simulink model "lss"  (R2022b)
settings: Solver=FixedStepAuto  StartTime=0.0  StopTime=Inf  FixedStep=0.001  RelTol=1e-3  EnableMultiTasking=on
InitFcn:
  | clear mex
model workspace (MAT data in the model file):
  worldsim_instance : object (value not decoded)
values from neighbouring files (symbols this model uses):
  ADAS_Control_Mode = 1    [LSS_parameters.m]    (also in lss_ini_param.sldd = 1.0)
  butter_a = 1.0 -1.9911142922016536 0.99115359586893548    [lss_ini_param.sldd]
  butter_a_lka_out = 1.0 -1.5610180758007179 0.641351538057563    [lss_ini_param.sldd]
  butter_b = 9.825916820482009E-6 1.9651833640964018E-5 9.825916820482009E-6    [lss_ini_param.sldd]
  butter_b_lka_out = 0.020083365564211246 0.040166731128422492 0.020083365564211246    [lss_ini_param.sldd]
  index_variant_approaching_speed = 3.0    [lss_ini_param.sldd]
  initCond = vi_worldsim_load_scenario(worldsim_process,scenario_path,'lss_online')    [launcher.m]
  LDW_Activity_Flag = 1    [LSS_parameters.m]    (also in lss_ini_param.sldd = 1.0)
  LDW_Freq_Hz = Sensor_Freq_worldsim    [LSS_parameters.m]    (also in lss_ini_param.sldd = 50.0)
  LDW_LaneGap_dydt_Warning = 50    [LSS_parameters.m]    (also in lss_ini_param.sldd = 50.0)
  LDW_LaneGap_Warning = [0.5 0.25]    [LSS_parameters.m]    (also in lss_ini_param.sldd = 0.5 0.25)
  LDW_Min_Speed = 60    [LSS_parameters.m]    (also in lss_ini_param.sldd = 60.0)
  LDW_Steer_Vibration_Amplitude = 5    [LSS_parameters.m]    (also in lss_ini_param.sldd = 5.0)
  LDW_Steer_Vibration_Freq = 25    [LSS_parameters.m]    (also in lss_ini_param.sldd = 25.0)
  LKA_Activity_Flag = 1    [LSS_parameters.m]    (also in lss_ini_param.sldd = 1.0)
  LKA_D = [0.2 0.3]    [LSS_parameters.m]    (also in lss_ini_param.sldd = 0.2 0.3)
  LKA_Dyn_Rate_Limiter_Gain = 0.1    [LSS_parameters.m]    (also in lss_ini_param.sldd)
  LKA_Dyn_Rate_Limiter_Power = 10    [LSS_parameters.m]    (also in lss_ini_param.sldd = 10.0)
  LKA_Error_dydt_Off = 1    [LSS_parameters.m]    (also in lss_ini_param.sldd = 1.0)
  LKA_Error_Max = 3    [LSS_parameters.m]    (also in lss_ini_param.sldd = 3.0)
  LKA_Error_Off = 0.5    [LSS_parameters.m]    (also in lss_ini_param.sldd)
  LKA_Freq_Hz = Sensor_Freq_worldsim    [LSS_parameters.m]    (also in lss_ini_param.sldd = 50.0)
  LKA_I = [0.025 0.05]    [LSS_parameters.m]    (also in lss_ini_param.sldd = 0.025 0.05)
  LKA_Lane_Gap_Activate = [0.25 0.125]    [LSS_parameters.m]    (also in lss_ini_param.sldd = -0.05 0.125)
  LKA_Lane_Gap_dydt_Activate = 50    [LSS_parameters.m]    (also in lss_ini_param.sldd = 50.0)
  LKA_Min_Speed = 60    [LSS_parameters.m]    (also in lss_ini_param.mat = 50; lss_ini_param.sldd = 50.0)
  LKA_On_Display_Freq = 5    [LSS_parameters.m]    (also in lss_ini_param.sldd = 5.0)
  LKA_P = [0.1 0.2]    [LSS_parameters.m]    (also in lss_ini_param.sldd = 0.1 0.2)
  LKA_Steer_Rate_Max_radps = 1    [LSS_parameters.m]    (also in lss_ini_param.sldd = 1.0)
  radar_source = 2    [LSS_parameters.m]    (also in lss_ini_param.sldd = 2.0)
  Sensor_Freq_worldsim = 50    [launcher.m]    (also in lss_ini_param.sldd = 50.0)
  simulation_crt = '../VI-CarRealTime_model/SedanCar_WorldSim_Offline_send_svm.xml'    [launcher.m]
  stop_number_collisions = 5    [launcher.m]
  stop_speed = 0.001    [launcher.m]
  stop_time = 20    [launcher.m]
  target_speed = 72    [LSS_parameters.m]    (also in launcher.m = initCond.initialVelocity * 3.6)
  variant_approaching_speed = v_lat    [launcher.m]    (also in lss_ini_param.sldd = 0.2 0.3 0.4 0.5 0.6)
  vehicle_width = 1.86    [LSS_parameters.m]    (also in lss_ini_param.sldd = 2.05)
undefined symbols (not defined in the file or in its folder): Driver_Demands, light_brake_center, light_brake_left, light_brake_right, steer_assist, vicrt_initcallback, vicrt_initmexcallback, vicrt_simulationmanager
libraries: simulink x39, simwbSfunlib x15, viworldsim_lib x5
(part 2 of 6)

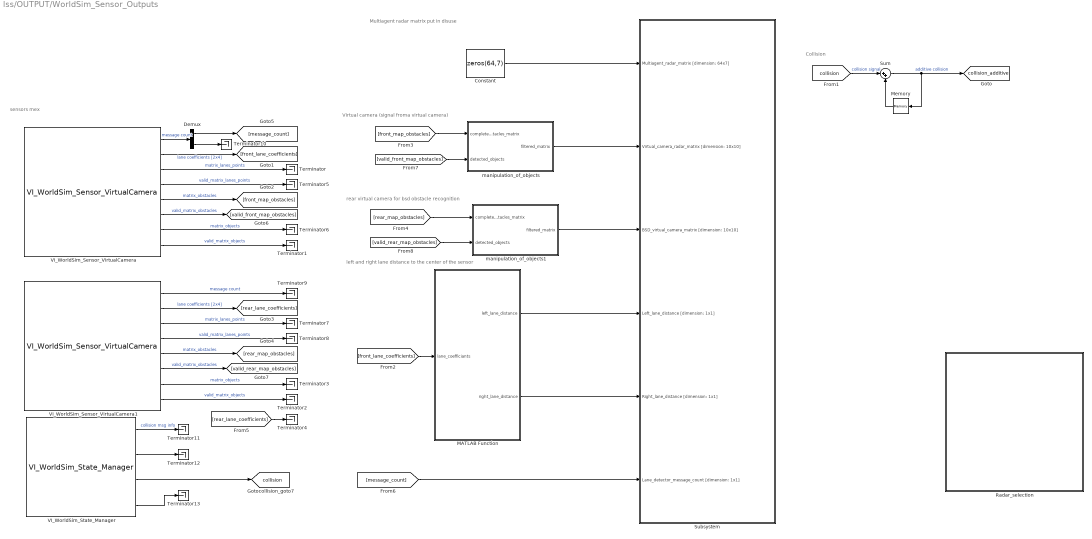
== system lss/OUTPUT/WorldSim_Sensor_Outputs ==
  note: Collision
  note: left and right lane distance to the center of the sensor
  note: Virtual camera (signal froma virtual camera)
  note: Multiagent radar matrix
      | put in disuse
  note: rear virtual camera for bsd obstacle recognition
  note: sensors mex
  Constant : Constant  Value=zeros(64,7)
  Demux : Demux  Outputs=2
  MATLAB Function : MATLAB Function  TreatAsAtomicUnit=on
  Memory : Memory  InheritSampleTime=on
  Radar_selection : Subsystem
  Subsystem : Subsystem
  Sum : Sum  Inputs=|++
  Terminator{,1..13} (14 alike) : Terminator
  VI_WorldSim_Sensor_VirtualCamera : viworldsim_lib/VI-WorldSim Sensors/VI_WorldSim_Sensor_VirtualCamera  worldsim_endpoint_ip=worldsim_instance.endpoint_ip  worldsim_endpoint_port=worldsim_instance.endpoint_port  worldsim_car_name='ego'  worldsim_sensor_name='Front_VirtualCam'  max_lanes=10  max_obstacles=10  worldsim_verbose=off
  VI_WorldSim_Sensor_VirtualCamera1 : viworldsim_lib/VI-WorldSim Sensors/VI_WorldSim_Sensor_VirtualCamera  worldsim_endpoint_ip=worldsim_instance.endpoint_ip  worldsim_endpoint_port=worldsim_instance.endpoint_port  worldsim_car_name='ego'  worldsim_sensor_name='Rear_VirtualCam'  max_lanes=10  max_obstacles=10  worldsim_verbose=off
  VI_WorldSim_State_Manager : viworldsim_lib/VI-WorldSim Sensors/VI_WorldSim_State_Manager  worldsim_endpoint_ip=worldsim_instance.endpoint_ip  worldsim_endpoint_port=worldsim_instance.endpoint_port  worldsim_car_name='ego'  worldsim_verbose=off
  manipulation_of_objects : MATLAB Function  TreatAsAtomicUnit=on
  manipulation_of_objects1 : MATLAB Function  TreatAsAtomicUnit=on
  tag scope: collision=global, collision_additive=global
  wires:
  Sum/1 -> Memory/1, [collision_additive]  "additive collision"
  [collision] -> Sum/1  "collision signal"
  Memory/1 -> Sum/2
  MATLAB Function/1(left_lane_distance) -> Subsystem/4(Left_lane_distance [dimension: 1x1])
  [message_count] -> Subsystem/6(Lane_detector_message_count [dimension: 1x1])
  manipulation_of_objects1/1(filtered_matrix) -> Subsystem/3(BSD_virtual_camera_matrix [dimension: 10x10])
  manipulation_of_objects/1(filtered_matrix) -> Subsystem/2(Virtual_camera_radar_matrix [dimension: 10x10])
  Constant/1 -> Subsystem/1(Multiagent_radar_matrix [dimension: 64x7])
  [valid_rear_map_obstacles] -> manipulation_of_objects1/2(detected_objects)
  MATLAB Function/2(right_lane_distance) -> Subsystem/5(Right_lane_distance [dimension: 1x1])
  [front_lane_coefficients] -> MATLAB Function/1(lane_coefficiants)
  [rear_map_obstacles] -> manipulation_of_objects1/1(complete_obstacles_matrix)
  [valid_front_map_obstacles] -> manipulation_of_objects/2(detected_objects)
  [front_map_obstacles] -> manipulation_of_objects/1(complete_obstacles_matrix)
  VI_WorldSim_Sensor_VirtualCamera/1 -> Demux/1  "message count"
  VI_WorldSim_State_Manager/1 -> Terminator11/1  "collision msg info"
  VI_WorldSim_Sensor_VirtualCamera/8 -> Terminator1/1  "valid_matrix_objects"
  VI_WorldSim_Sensor_VirtualCamera/5 -> [front_map_obstacles]  "matrix_obstacles"
  VI_WorldSim_Sensor_VirtualCamera/4 -> Terminator5/1  "valid_matrix_lanes_points"
  VI_WorldSim_Sensor_VirtualCamera/6 -> [valid_front_map_obstacles]  "valid_matrix_obstacles"
  VI_WorldSim_Sensor_VirtualCamera1/2 -> [rear_lane_coefficients]  "lane coefficients [2x4]"
  VI_WorldSim_Sensor_VirtualCamera/3 -> Terminator/1  "matrix_lanes_points"
  VI_WorldSim_Sensor_VirtualCamera1/1 -> Terminator9/1  "message count"
  VI_WorldSim_Sensor_VirtualCamera1/7 -> Terminator3/1  "matrix_objects"
  VI_WorldSim_Sensor_VirtualCamera1/8 -> Terminator2/1  "valid_matrix_objects"
  VI_WorldSim_Sensor_VirtualCamera/7 -> Terminator6/1  "matrix_objects"
  VI_WorldSim_Sensor_VirtualCamera/2 -> [front_lane_coefficients]  "lane coefficients [2x4]"
  VI_WorldSim_Sensor_VirtualCamera1/4 -> Terminator8/1  "valid_matrix_lanes_points"
  VI_WorldSim_State_Manager/3 -> [collision]
  VI_WorldSim_Sensor_VirtualCamera1/3 -> Terminator7/1  "matrix_lanes_points"
  [rear_lane_coefficients] -> Terminator4/1
  Demux/2 -> Terminator10/1
  VI_WorldSim_Sensor_VirtualCamera1/5 -> [rear_map_obstacles]  "matrix_obstacles"
  VI_WorldSim_Sensor_VirtualCamera1/6 -> [valid_rear_map_obstacles]  "valid_matrix_obstacles"
  Demux/1 -> [message_count]
  VI_WorldSim_State_Manager/2 -> Terminator12/1
  VI_WorldSim_State_Manager/4 -> Terminator13/1

== system lss/OUTPUT/rough data reporting ==
  Cast To Double : DataTypeConversion  OutDataTypeStr=double  SaturateOnIntegerOverflow=off  RndMeth=Floor
  Cast To Double1 : DataTypeConversion  OutDataTypeStr=double  SaturateOnIntegerOverflow=off  RndMeth=Floor
  Clock : Clock
  Compare To Constant : simulink/Logic and Bit Operations/Compare To Constant  relop=<=  const=0.0  OutDataTypeStr=boolean
  Compare To Constant1 : simulink/Logic and Bit Operations/Compare To Constant  relop=<=  const=0.0  OutDataTypeStr=boolean
  Compare To Constant2 : simulink/Logic and Bit Operations/Compare To Constant  relop=>  const=0.1  OutDataTypeStr=boolean
  Product : Product
  Scope LDW_Steering_Torque_in_out : Scope  NumInputPorts=2
  Sum1 : Sum
  To Workspace : ToWorkspace  VariableName=number_collision  SampleTime=-1
      settings: Save2DSignal=2-D array (concatenate along first dimension)
  To Workspace1 : ToWorkspace  VariableName=longitudinal_accelerations  SampleTime=-1
      settings: Save2DSignal=2-D array (concatenate along first dimension)
  To Workspace2 : ToWorkspace  VariableName=lateral_accelerations  SampleTime=-1
      settings: Save2DSignal=2-D array (concatenate along first dimension)
  To Workspace3 : ToWorkspace  VariableName=crossed_lanes  SampleTime=-1
      settings: Save2DSignal=2-D array (concatenate along first dimension)
  wires:
  Clock/1 -> Compare To Constant2/1
  Compare To Constant1/1 -> Cast To Double1/1
  [Lateral_Accelerations] -> To Workspace2/1
  [LaneGap_right_ws] -> Compare To Constant1/1
  Cast To Double/1 -> Sum1/1
  Compare To Constant2/1 -> Product/2
  [collision_additive] -> To Workspace/1
  Compare To Constant/1 -> Cast To Double/1
  [Longitudinal_Accelerations] -> To Workspace1/1
  [LaneGap_left_ws] -> Compare To Constant/1
  Product/1 -> To Workspace3/1
  Cast To Double1/1 -> Sum1/2
  Sum1/1 -> Product/1
  [Steering_feedback_torque] -> Scope LDW_Steering_Torque_in_out/2  "Output Steering Wheel Torque"
  [LDW_Steering_Torque] -> Scope LDW_Steering_Torque_in_out/1  "LDW Additional Steering Assist torque"

== system lss/VI-CarRealTime/Input_Bus ==
  Driver_Demands.str_swa : Inport
  steer_assist.torque : Inport  Port=2
  Driver_Demands.throttle : Inport  Port=3
  Driver_Demands.clutch : Inport  Port=4
  Driver_Demands.brake : Inport  Port=5
  Driver_Demands.gear : Inport  Port=6
  Bus2Map : Subsystem
  Inputs : Subsystem
  VicrtBusAssignment : BusAssignment  AssignedSignals=Driver_Demands.str_swa,steer_assist.torque,Driver_Demands.throttle,Driver_Demands.clutch,Driver_Demands.brake,Driver_Demands.gear
  vicrt input : Outport
  wires:
  Bus2Map/1(Map Out) -> vicrt input/1
  VicrtBusAssignment/1 -> Bus2Map/1(Bus In)
  Inputs/1(Inputs) -> VicrtBusAssignment/1  "Inputs"
  Driver_Demands.str_swa/1 -> VicrtBusAssignment/2
  steer_assist.torque/1 -> VicrtBusAssignment/3
  Driver_Demands.throttle/1 -> VicrtBusAssignment/4
  Driver_Demands.clutch/1 -> VicrtBusAssignment/5
  Driver_Demands.brake/1 -> VicrtBusAssignment/6
  Driver_Demands.gear/1 -> VicrtBusAssignment/7

== system lss/VI-CarRealTime/Output_Bus ==
  Outputs : Inport
  IOmap2bus : Subsystem
  VicrtBusSelector : BusSelector  OutputSignals=aero_forces,Brake,bul_jounce_stop_data,bul_rebound_stop_data,bur_jounce_stop_data,bur_rebound_stop_data,bus_dmp_jounce_stop_data,bus_ins_jounce_stop_data,bus_roll_dmp_jounce_stop_data,bus_spr_jounce_stop_data,chassis_accelerations,chassis_displacements,chassis_velocities,clutch,condition_sensors,cross_weight,dal_ride_damper_data,Damper,dar_ride_damper_data,das_ride_damper_data,das_roll_damper_data,das_third_damper_data,differential_central,differential_front,differential_rear,differential_speeds,differential_torques,driver_demands,driving_machine_monitor,engine,fuel_consumption,ges_chassis_XFORM,Gyro,Hook_rear,Inerter,inl_ride_inerter_data,inr_ride_inerter_data,ins_inerter_data,jfs_torsional_stiffness_data,Jounce_Bumper,nsl_ride_spring_data,nsr_ride_spring_data,nss_ride_spring_data,Rebound_Bumper,res_dmp_rebound_stop_data,res_ins_rebound_stop_data,res_roll_dmp_rebound_stop_data,res_spr_rebound_stop_data,rhl_front_setup_sensor_data,rhl_rear_setup_sensor_data,rhr_front_setup_sensor_data,rhr_rear_setup_sensor_data,rhs_front_setup_sensor_data,rhs_rear_setup_sensor_data,Road,Sensor,Spring,Steering_System,Suspension,System,System_Mass_Center,til_wheel_tire_forces,til_wheel_tire_kinematics,til_wheel_tire_rolling_states,Tire,tir_wheel_tire_forces,tir_wheel_tire_kinematics,tir_wheel_tire_rolling_states,torque_converter,transmission,ues_third_spring_data,upright_accelerometer,Vehicle,Vehicle_States,Wheel,wheel_angles,whl_front_wheel_XFORM,whl_rear_wheel_XFORM,whl_twin_rear_wheel_XFORM,whr_front_wheel_XFORM,whr_rear_wheel_XFORM,whr_twin_rear_wheel_XFORM,Steering_Column,Steering_Torsion_Bar,Steering_Rack_Pinion,Motor,path_sensor,Animator_Widget,ges_hub_XFORMFL,hub2cp_XFORMFL,cp_force_longitudinalFL,cp_force_lateralFL,cp_force_normalFL,ges_hub_XFORMFR,hub2cp_XFORMFR,cp_force_longitudinalFR,cp_force_lateralFR,cp_force_normalFR,ges_hub_XFORMRL,hub2cp_XFORMRL,cp_force_longitudinalRL,cp_force_lateralRL,cp_force_normalRL,ges_hub_XFORMRR,hub2cp_XFORMRR,cp_force_longitudinalRR,cp_force_lateralRR,cp_force_normalRR,Road_Material  OutputAsBus=on
  adapter : Subsystem
  OutputBus : Outport  VectorParamsAs1DForOutWhenUnconnected=off
  wires:
  IOmap2bus/1(Out) -> VicrtBusSelector/1
  Outputs/1 -> IOmap2bus/1(In)
  VicrtBusSelector/1 -> adapter/1(inputBus)
  adapter/1(outputBus) -> OutputBus/1

== system lss/VI-CarRealTime/vicrt_mex Standard ==
  In1 : Inport
  vicrt_mex : S-Function  InitFcn=vicrt_initmexcallback(gcb);  FunctionName=vicrt_mex  Parameters=vicrt_inputfile,vicrt_outprefix,AniFlag,intStep,inpPortDim,outPortDim,NoDirectFeedthrough,AuxDataStruct,inpPortVecSize,outPortVecSize  SFunctionDeploymentMode=off  EnableBusSupport=off
  Out1 : Outport
  wires:
  In1/1 -> vicrt_mex/1
  vicrt_mex/1 -> Out1/1

== system lss/VI-WorldSim Lights Manager/Lights ==
  light_brake_left : Inport
  light_brake_right : Inport  Port=2
  light_brake_center : Inport  Port=3
  Bus Selector : BusSelector  OutputSignals=light_low_beam_left,light_low_beam_right,light_high_beam_left,light_high_beam_right,light_indicator_left,light_indicator_right,light_fog_left,light_fog_right,light_tail_left,light_tail_right,light_brake_left,light_brake_right,light_brake_center,light_reverse,light_daytime
  Default Lights Bus : Subsystem
  LightsBusAssignment : BusAssignment  AssignedSignals=light_brake_left,light_brake_right,light_brake_center
  Mux : Mux  Inputs=15
  Out1 : Outport  VectorParamsAs1DForOutWhenUnconnected=off
  wires:
  LightsBusAssignment/1 -> Bus Selector/1
  Bus Selector/5 -> Mux/5  "<light_indicator_left>"
  Default Lights Bus/1(Out1) -> LightsBusAssignment/1
  Bus Selector/11 -> Mux/11  "<light_brake_left>"
  Bus Selector/10 -> Mux/10  "<light_tail_right>"
  Bus Selector/2 -> Mux/2  "<light_low_beam_right>"
  Bus Selector/9 -> Mux/9  "<light_tail_left>"
  Bus Selector/12 -> Mux/12  "<light_brake_right>"
  Mux/1 -> Out1/1
  Bus Selector/8 -> Mux/8  "<light_fog_right>"
  Bus Selector/14 -> Mux/14  "<light_reverse>"
  Bus Selector/4 -> Mux/4  "<light_high_beam_right>"
  Bus Selector/3 -> Mux/3  "<light_high_beam_left>"
  Bus Selector/15 -> Mux/15  "<light_daytime>"
  Bus Selector/13 -> Mux/13  "<light_brake_center>"
  Bus Selector/6 -> Mux/6  "<light_indicator_right>"
  Bus Selector/1 -> Mux/1  "<light_low_beam_left>"
  Bus Selector/7 -> Mux/7  "<light_fog_left>"
  light_brake_left/1 -> LightsBusAssignment/2
  light_brake_right/1 -> LightsBusAssignment/3
  light_brake_center/1 -> LightsBusAssignment/4

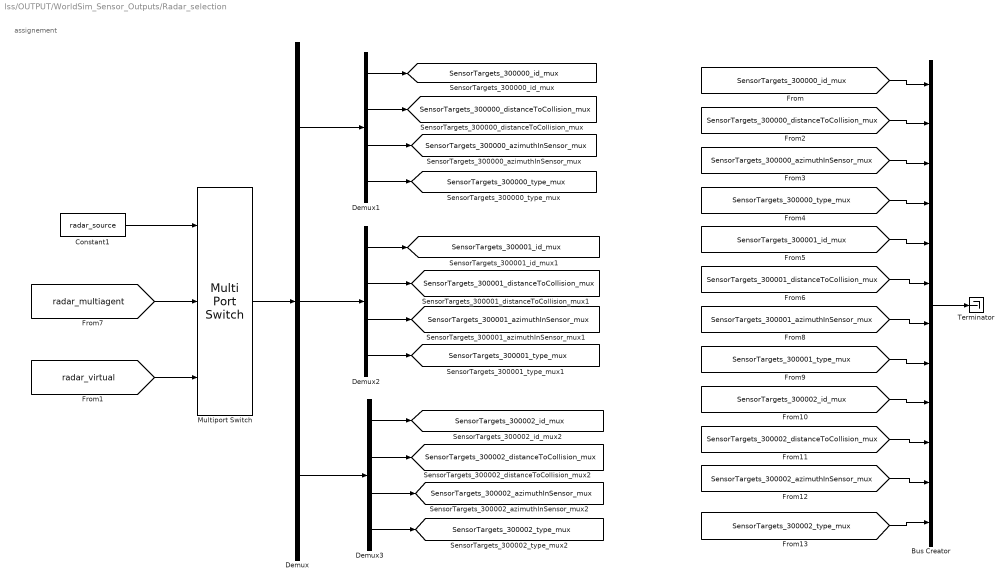
== system lss/OUTPUT/WorldSim_Sensor_Outputs/Radar_selection ==
  note: assignement
  Bus Creator : BusCreator  Inputs=12
  Constant1 : Constant  Value=radar_source
  Demux : Demux  Outputs=3
  Demux1 : Demux
  Demux2 : Demux
  Demux3 : Demux
  Multiport Switch : MultiPortSwitch  Inputs=2  SaturateOnIntegerOverflow=off  InputSameDT=off
  Terminator : Terminator
  tag scope: SensorTargets_300000_azimuthInSensor_mux=global, SensorTargets_300000_distanceToCollision_mux=global, SensorTargets_300000_id_mux=global, SensorTargets_300000_type_mux=global, SensorTargets_300001_azimuthInSensor_mux=global, SensorTargets_300001_distanceToCollision_mux=global, SensorTargets_300001_id_mux=global, SensorTargets_300001_type_mux=global, SensorTargets_300002_azimuthInSensor_mux=global, SensorTargets_300002_distanceToCollision_mux=global, SensorTargets_300002_id_mux=global, SensorTargets_300002_type_mux=global
  wires:
  [radar_virtual] -> Multiport Switch/3
  [radar_multiagent] -> Multiport Switch/2
  Constant1/1 -> Multiport Switch/1
  Multiport Switch/1 -> Demux/1
  Demux1/1 -> [SensorTargets_300000_id_mux]
  Demux3/4 -> [SensorTargets_300002_type_mux]
  Demux3/1 -> [SensorTargets_300002_id_mux]
  Demux1/4 -> [SensorTargets_300000_type_mux]
  Demux3/2 -> [SensorTargets_300002_distanceToCollision_mux]
  Demux2/3 -> [SensorTargets_300001_azimuthInSensor_mux]
  Demux1/2 -> [SensorTargets_300000_distanceToCollision_mux]
  Demux/1 -> Demux1/1
  Demux1/3 -> [SensorTargets_300000_azimuthInSensor_mux]
  Demux2/2 -> [SensorTargets_300001_distanceToCollision_mux]
  Demux3/3 -> [SensorTargets_300002_azimuthInSensor_mux]
  Demux2/4 -> [SensorTargets_300001_type_mux]
  Demux/3 -> Demux3/1
  Demux/2 -> Demux2/1
  Demux2/1 -> [SensorTargets_300001_id_mux]
  [SensorTargets_300000_id_mux] -> Bus Creator/1
  [SensorTargets_300000_distanceToCollision_mux] -> Bus Creator/2
  [SensorTargets_300000_azimuthInSensor_mux] -> Bus Creator/3
  [SensorTargets_300000_type_mux] -> Bus Creator/4
  [SensorTargets_300001_id_mux] -> Bus Creator/5
  [SensorTargets_300001_distanceToCollision_mux] -> Bus Creator/6
  [SensorTargets_300001_azimuthInSensor_mux] -> Bus Creator/7
  [SensorTargets_300001_type_mux] -> Bus Creator/8
  [SensorTargets_300002_id_mux] -> Bus Creator/9
  [SensorTargets_300002_distanceToCollision_mux] -> Bus Creator/10
  [SensorTargets_300002_azimuthInSensor_mux] -> Bus Creator/11
  [SensorTargets_300002_type_mux] -> Bus Creator/12
  Bus Creator/1 -> Terminator/1

== system lss/OUTPUT/WorldSim_Sensor_Outputs/Subsystem ==
  Multiagent_radar_matrix [dimension: 64x7] : Inport
  Virtual_camera_radar_matrix [dimension: 10x10] : Inport  Port=2
  BSD_virtual_camera_matrix [dimension: 10x10] : Inport  Port=3
  Left_lane_distance [dimension: 1x1] : Inport  Port=4
  Right_lane_distance [dimension: 1x1] : Inport  Port=5
  Lane_detector_message_count [dimension: 1x1] : Inport  Port=6
  Semitrack : Constant  Value=vehicle_width/2
  Terminator : Terminator
  Terminator1 : Terminator
  bsd setection from ostacle recognition : Subsystem
  lane marking acquisition : Subsystem
  "multiagent radar SimpleRadar_... are single double representing id, yaw, range, power_db, range_rate, yaw_rate, status" : Subsystem
  "obstacle detection " : Subsystem
  tag scope: frame_worldsim_left=global, frame_worldsim_right=global
  wires:
  Semitrack/1 -> lane marking acquisition/1(Semitrack), bsd setection from ostacle recognition/1(semitrack)
  Virtual_camera_radar_matrix [dimension: 10x10]/1 -> "obstacle detection "/1(Virtual_camera_obstacle_matrix)
  BSD_virtual_camera_matrix [dimension: 10x10]/1 -> bsd setection from ostacle recognition/2(BSD_matrix_obstalces)
  Left_lane_distance [dimension: 1x1]/1 -> lane marking acquisition/2(Left_lane_marking)
  Right_lane_distance [dimension: 1x1]/1 -> lane marking acquisition/3(Right_lane_marking)
  Multiagent_radar_matrix [dimension: 64x7]/1 -> "multiagent radar SimpleRadar_... are single double representing id, yaw, range, power_db, range_rate, yaw_rate, status"/1(Virtual_radar_obstacle_matrix)
  Lane_detector_message_count [dimension: 1x1]/1 -> [frame_worldsim_right], [frame_worldsim_left]
  [frame_worldsim_left] -> Terminator/1
  [frame_worldsim_right] -> Terminator1/1

== system lss/VI-CarRealTime/Input_Bus/Bus2Map ==
  Bus In : Inport
  Bus Selector : BusSelector  OutputSignals=Driver_Demands.str_swa,Subsystem_Activation.Internal_Steering_Column_Activity,Driver_Demands.rack_displacement,Driver_Demands.throttle,Driver_Demands.gear,Driver_Demands.clutch,Driver_Demands.brake,Driver_Demands.target_speed,Driver_Demands.target_acc,Brake_System_General.brk_mast_cyl_pres,Brake_System_General.brk_bias_front,ABS.Internal_ABS_Activity,ABS.ABS_threshold,Driver_Demands.user_maneuver_ID,Driver_Demands.user_input_steering,Driver_Demands.user_input_throttle,Driver_Demands.user_input_braking,Driver_Demands.user_input_gear,Driver_Demands.user_input_clutch,TCS.Internal_TCS_Activity,TCS.TCS_threshold,Friction.tire_mu.L1,Friction.tire_mu.L2,Friction.tire_mu.R1,Friction.tire_mu.R2,Subsystem_Activation.Internal_Brake_System_Activity.L1,Brake_System.brk_mmag_sign.L1,Brake_System.brk_mmag_unsign.L1,Brake_System.brk_pres.L1,Brake_System.brk_pres_gain.L1,Brake_System.brk_mu.L1,Subsystem_Activation.Internal_Brake_System_Activity.L2,Brake_System.brk_mmag_sign.L2,Brake_System.brk_mmag_unsign.L2,Brake_System.brk_pres.L2,Brake_System.brk_pres_gain.L2,Brake_System.brk_mu.L2,Subsystem_Activation.Internal_Brake_System_Activity.R1,Brake_System.brk_mmag_sign.R1,Brake_System.brk_mmag_unsign.R1,Brake_System.brk_pres.R1,Brake_System.brk_pres_gain.R1,Brake_System.brk_mu.R1,Subsystem_Activation.Internal_Brake_System_Activity.R2,Brake_System.brk_mmag_sign.R2,Brake_System.brk_mmag_unsign.R2,Brake_System.brk_pres.R2,Brake_System.brk_pres_gain.R2,Brake_System.brk_mu.R2,Hook.Fx.rear,Hook.Fy.rear,Hook.Fz.rear,Hook.Mx.rear,Hook.My.rear,Hook.Mz.rear,Rear_Steering_Actuator_disp.str_swa.left,Rear_Steering_Actuator_disp.str_swa.right,Steering.steer_at_spindle.L1,Steering.steer_at_spindle.L2,Steering.steer_at_spindle.R1,Steering.steer_at_spindle.R2,Steering.Internal_Hand_Wheel_Torque_Computation,Steering.Hand_Wheel_Torque,Subsystem_Activation.Internal_Clutch_Activity,Subsystem_Activation.Internal_Engine_Activity,Subsystem_Activation.Internal_Engine_Idle_MaxRev_Controls_Activity,Subsystem_Activation.Internal_Gearbox_Activity,Subsystem_Activation.Internal_CentralDifferential_Activity,Subsystem_Activation.Internal_FrontDifferential_Activity,Subsystem_Activation.Internal_RearDifferential_Activity,Engine.engine_omega,Engine.engine_max_trq,Engine.engine_min_trq,Engine.engine_trq,Engine.clutch_inputplate_torque,Engine.non_termic_engine_trq,Engine.efficiency,Engine.throttle_scaling,Engine.control_mode,Engine.throttle_offset,Clutch.clutch_trq,Clutch.gearbox_inputshaft_torque,Clutch.inputplate_angle,Clutch.inputplate_omega,Clutch.inputplate_alpha,Clutch.efficiency,Differential_Central.efficiency,Differential_Central.diff_front_inputshaft_torque,Differential_Central.diff_rear_inputshaft_torque,Differential_Central.gearbox_outputshaft_angle,Differential_Central.gearbox_outputshaft_omega,Differential_Central.gearbox_outputshaft_alpha,Differential_Front.efficiency,Differential_Front.wheel_front_left_torque,Differential_Front.wheel_front_right_torque,Differential_Front.diff_central_front_outputshaft_angle,Differential_Front.diff_central_front_outputshaft_omega,Differential_Front.diff_central_front_outputshaft_alpha,Differential_Rear.efficiency,Differential_Rear.wheel_rear_left_torque,Differential_Rear.wheel_rear_right_torque,Differential_Rear.diff_central_rear_outputshaft_angle,Differential_Rear.diff_central_rear_outputshaft_omega,Differential_Rear.diff_central_rear_outputshaft_alpha,Antiroll_Bar.activity_flag.front,Antiroll_Bar.activity_flag.rear,Antiroll_Bar.force.front,Antiroll_Bar.force.rear,Wheel_driving.moment.L1,Wheel_driving.moment.L2,Wheel_driving.moment.R1,Wheel_driving.moment.R2,Subsystem_Activation.Internal_Aero_Activity,Aerodynamic.my_scaling,Aerodynamic.fx_central_scaling,Aerodynamic.fz_front_scaling,Aerodynamic.fz_rear_scaling,Aerodynamic.fx_front,Aerodynamic.fy_front,Aerodynamic.fz_front,Aerodynamic.fx_rear,Aerodynamic.fy_rear,Aerodynamic.fz_rear,Aerodynamic.fx_center,Aerodynamic.fy_center,Aerodynamic.fz_center,Aerodynamic.mx,Aerodynamic.my,Aerodynamic.mz,Irregularity.road.L1,Irregularity.road.L2,Irregularity.road.R1,Irregularity.road.R2,Main_Damper.force.L1,Main_Damper.activity_flag.L1,Main_Damper.force.L2,Main_Damper.activity_flag.L2,Main_Damper.force.R1,Main_Damper.activity_flag.R1,Main_Damper.force.R2,Main_Damper.activity_flag.R2,Main_Spring.force.L1,Main_Spring.activity_flag.L1,Main_Spring.force.L2,Main_Spring.activity_flag.L2,Main_Spring.force.R1,Main_Spring.activity_flag.R1,Main_Spring.force.R2,Main_Spring.activity_flag.R2,Main_Bumpstop.force.L1,Main_Bumpstop.activity_flag.L1,Main_Bumpstop.force.L2,Main_Bumpstop.activity_flag.L2,Main_Bumpstop.force.R1,Main_Bumpstop.activity_flag.R1,Main_Bumpstop.force.R2,Main_Bumpstop.activity_flag.R2,Main_Reboundstop.force.L1,Main_Reboundstop.activity_flag.L1,Main_Reboundstop.force.L2,Main_Reboundstop.activity_flag.L2,Main_Reboundstop.force.R1,Main_Reboundstop.activity_flag.R1,Main_Reboundstop.force.R2,Main_Reboundstop.activity_flag.R2,Auxiliary_vertical.force.L1,Auxiliary_vertical.activity_flag.L1,Auxiliary_vertical.force.L2,Auxiliary_vertical.activity_flag.L2,Auxiliary_vertical.force.R1,Auxiliary_vertical.activity_flag.R1,Auxiliary_vertical.force.R2,Auxiliary_vertical.activity_flag.R2,Main_Inerter.force.L1,Main_Inerter.activity_flag.L1,Main_Inerter.force.L2,Main_Inerter.activity_flag.L2,Main_Inerter.force.R1,Main_Inerter.activity_flag.R1,Main_Inerter.force.R2,Main_Inerter.activity_flag.R2,Third_Element.Damper_force.front,Third_Element.Damper_activity_flag.front,Third_Element.Damper_force.rear,Third_Element.Damper_activity_flag.rear,Third_Element.Spring.front,Third_Element.Spring_activity_flag.front,Third_Element.Spring.rear,Third_Element.Spring_activity_flag.rear,Mono_Element.Damper.front,Mono_Element.Damper_activity_flag.front,Mono_Element.Damper.rear,Mono_Element.Damper_activity_flag.rear,Mono_Element.Inerter.front,Mono_Element.Inerter_activity_flag.front,Mono_Element.Inerter.rear,Mono_Element.Inerter_activity_flag.rear,Mono_Element.Spring.front,Mono_Element.Spring_activity_flag.front,Mono_Element.Spring.rear,Mono_Element.Spring_activity_flag.rear,Mono_Element.Bumpstop_Spring.front,Mono_Element.Bumpstop_Spring_activity_flag.front,Mono_Element.Bumpstop_Spring.rear,Mono_Element.Bumpstop_Spring_activity_flag.rear,Mono_Element.Reboundstop_Spring.front,Mono_Element.Reboundstop_Spring_activity_flag.front,Mono_Element.Reboundstop_Spring.rear,Mono_Element.Reboundstop_Spring_activity_flag.rear,Mono_Element.Bumpstop_Damper.front,Mono_Element.Bumpstop_Damper_activity_flag.front,Mono_Element.Bumpstop_Damper.rear,Mono_Element.Bumpstop_Damper_activity_flag.rear,Mono_Element.Reboundstop_Damper.front,Mono_Element.Reboundstop_Damper_activity_flag.front,Mono_Element.Reboundstop_Damper.rear,Mono_Element.Reboundstop_Damper_activity_flag.rear,Mono_Element.Roll_Damper.front,Mono_Element.Roll_Damper_activity_flag.front,Mono_Element.Roll_Damper.rear,Mono_Element.Roll_Damper_activity_flag.rear,Subsystem_Activation.Tire_Force_x.L1,Subsystem_Activation.Tire_Force_y.L1,Subsystem_Activation.Tire_Force_z.L1,Subsystem_Activation.Tire_Moment_x.L1,Subsystem_Activation.Tire_Moment_y.L1,Subsystem_Activation.Tire_Moment_z.L1,Tire_Force.Fx.L1,Tire_Force.Fy.L1,Tire_Force.Fz.L1,Tire_Moment.Mx.L1,Tire_Moment.My.L1,Tire_Moment.Mz.L1,Subsystem_Activation.Tire_Force_x.L2,Subsystem_Activation.Tire_Force_y.L2,Subsystem_Activation.Tire_Force_z.L2,Subsystem_Activation.Tire_Moment_x.L2,Subsystem_Activation.Tire_Moment_y.L2,Subsystem_Activation.Tire_Moment_z.L2,Tire_Force.Fx.L2,Tire_Force.Fy.L2,Tire_Force.Fz.L2,Tire_Moment.Mx.L2,Tire_Moment.My.L2,Tire_Moment.Mz.L2,Subsystem_Activation.Tire_Force_x.R1,Subsystem_Activation.Tire_Force_y.R1,Subsystem_Activation.Tire_Force_z.R1,Subsystem_Activation.Tire_Moment_x.R1,Subsystem_Activation.Tire_Moment_y.R1,Subsystem_Activation.Tire_Moment_z.R1,Tire_Force.Fx.R1,Tire_Force.Fy.R1,Tire_Force.Fz.R1,Tire_Moment.Mx.R1,Tire_Moment.My.R1,Tire_Moment.Mz.R1,Subsystem_Activation.Tire_Force_x.R2,Subsystem_Activation.Tire_Force_y.R2,Subsystem_Activation.Tire_Force_z.R2,Subsystem_Activation.Tire_Moment_x.R2,Subsystem_Activation.Tire_Moment_y.R2,Subsystem_Activation.Tire_Moment_z.R2,Tire_Force.Fx.R2,Tire_Force.Fy.R2,Tire_Force.Fz.R2,Tire_Moment.Mx.R2,Tire_Moment.My.R2,Tire_Moment.Mz.R2,Ext_Body.force.X,Ext_Body.force.Y,Ext_Body.force.Z,Ext_Body.moment.X,Ext_Body.moment.Y,Ext_Body.moment.Z,Ext_Ground.force.X,Ext_Ground.force.Y,Ext_Ground.force.Z,Ext_Ground.moment.X,Ext_Ground.moment.Y,Ext_Ground.moment.Z,Ext_Tracking.force.X,Ext_Tracking.force.Y,Ext_Tracking.moment.X,Ext_Tracking.moment.Y,steer_assist.force,steer_assist.torque,steering_torque.torque,steering_assist.motor_torque,Steering_System.auxiliary_steering_torque,Steering_System.eps_map,Fuel_Mass.Internal_mass_activation,Fuel_Mass.External_mass,GearBox.efficiency,GearBox.transmission_ratio,GearBox.diff_central_inputshaft_torque,GearBox.clutch_outputplate_angle,GearBox.clutch_outputplate_omega,GearBox.clutch_outputplate_alpha,GearBox.automatic_gearbox_shifting_mode,GearBox.manual_shifting_activity,GearBox.sequential_shifting_activity,Driver_Demands.gear_upshift,Driver_Demands.gear_downshift
  Mux : Mux  Inputs=304
  Map Out : Outport
  wires:
  Mux/1 -> Map Out/1
  Bus In/1 -> Bus Selector/1
  Bus Selector/1 -> Mux/1  "<str_swa>"
  Bus Selector/2 -> Mux/2  "<Internal_Steering_Column_Activity>"
  Bus Selector/3 -> Mux/3  "<rack_displacement>"
  Bus Selector/4 -> Mux/4  "<throttle>"
  Bus Selector/5 -> Mux/5  "<gear>"
  Bus Selector/6 -> Mux/6  "<clutch>"
  Bus Selector/7 -> Mux/7  "<brake>"
  Bus Selector/8 -> Mux/8  "<target_speed>"
  Bus Selector/9 -> Mux/9  "<target_acc>"
  Bus Selector/10 -> Mux/10  "<brk_mast_cyl_pres>"
  Bus Selector/11 -> Mux/11  "<brk_bias_front>"
  Bus Selector/12 -> Mux/12  "<Internal_ABS_Activity>"
  Bus Selector/13 -> Mux/13  "<ABS_threshold>"
  Bus Selector/14 -> Mux/14  "<user_maneuver_ID>"
  Bus Selector/15 -> Mux/15  "<user_input_steering>"
  Bus Selector/16 -> Mux/16  "<user_input_throttle>"
  Bus Selector/17 -> Mux/17  "<user_input_braking>"
  Bus Selector/18 -> Mux/18  "<user_input_gear>"
  Bus Selector/19 -> Mux/19  "<user_input_clutch>"
  Bus Selector/20 -> Mux/20  "<Internal_TCS_Activity>"
  Bus Selector/21 -> Mux/21  "<TCS_threshold>"
  Bus Selector/22 -> Mux/22  "<L1>"
  Bus Selector/23 -> Mux/23  "<L2>"
  Bus Selector/24 -> Mux/24  "<R1>"
  Bus Selector/25 -> Mux/25  "<R2>"
  Bus Selector/26 -> Mux/26  "<L1>"
  Bus Selector/27 -> Mux/27  "<L1>"
  Bus Selector/28 -> Mux/28  "<L1>"
  Bus Selector/29 -> Mux/29  "<L1>"
  Bus Selector/30 -> Mux/30  "<L1>"
  Bus Selector/31 -> Mux/31  "<L1>"
  Bus Selector/32 -> Mux/32  "<L2>"
  Bus Selector/33 -> Mux/33  "<L2>"
  Bus Selector/34 -> Mux/34  "<L2>"
  Bus Selector/35 -> Mux/35  "<L2>"
  Bus Selector/36 -> Mux/36  "<L2>"
  Bus Selector/37 -> Mux/37  "<L2>"
  Bus Selector/38 -> Mux/38  "<R1>"
  Bus Selector/39 -> Mux/39  "<R1>"
  Bus Selector/40 -> Mux/40  "<R1>"
  Bus Selector/41 -> Mux/41  "<R1>"
  Bus Selector/42 -> Mux/42  "<R1>"
  Bus Selector/43 -> Mux/43  "<R1>"
  Bus Selector/44 -> Mux/44  "<R2>"
  Bus Selector/45 -> Mux/45  "<R2>"
  Bus Selector/46 -> Mux/46  "<R2>"
  Bus Selector/47 -> Mux/47  "<R2>"
  Bus Selector/48 -> Mux/48  "<R2>"
  Bus Selector/49 -> Mux/49  "<R2>"
  Bus Selector/50 -> Mux/50  "<rear>"
  Bus Selector/51 -> Mux/51  "<rear>"
  Bus Selector/52 -> Mux/52  "<rear>"
  Bus Selector/53 -> Mux/53  "<rear>"
  Bus Selector/54 -> Mux/54  "<rear>"
  Bus Selector/55 -> Mux/55  "<rear>"
  Bus Selector/56 -> Mux/56  "<left>"
  Bus Selector/57 -> Mux/57  "<right>"
  Bus Selector/58 -> Mux/58  "<L1>"
  Bus Selector/59 -> Mux/59  "<L2>"
  Bus Selector/60 -> Mux/60  "<R1>"
  Bus Selector/61 -> Mux/61  "<R2>"
  Bus Selector/62 -> Mux/62  "<Internal_Hand_Wheel_Torque_Computation>"
  Bus Selector/63 -> Mux/63  "<Hand_Wheel_Torque>"
  Bus Selector/64 -> Mux/64  "<Internal_Clutch_Activity>"
  Bus Selector/65 -> Mux/65  "<Internal_Engine_Activity>"
  Bus Selector/66 -> Mux/66  "<Internal_Engine_Idle_MaxRev_Controls_Activity>"
  Bus Selector/67 -> Mux/67  "<Internal_Gearbox_Activity>"
  Bus Selector/68 -> Mux/68  "<Internal_CentralDifferential_Activity>"
  Bus Selector/69 -> Mux/69  "<Internal_FrontDifferential_Activity>"
  Bus Selector/70 -> Mux/70  "<Internal_RearDifferential_Activity>"
  Bus Selector/71 -> Mux/71  "<engine_omega>"
  Bus Selector/72 -> Mux/72  "<engine_max_trq>"
  Bus Selector/73 -> Mux/73  "<engine_min_trq>"
  Bus Selector/74 -> Mux/74  "<engine_trq>"
  Bus Selector/75 -> Mux/75  "<clutch_inputplate_torque>"
  Bus Selector/76 -> Mux/76  "<non_termic_engine_trq>"
  Bus Selector/77 -> Mux/77  "<efficiency>"
  Bus Selector/78 -> Mux/78  "<throttle_scaling>"
  Bus Selector/79 -> Mux/79  "<control_mode>"
  Bus Selector/80 -> Mux/80  "<throttle_offset>"
  Bus Selector/81 -> Mux/81  "<clutch_trq>"
  Bus Selector/82 -> Mux/82  "<gearbox_inputshaft_torque>"
  Bus Selector/83 -> Mux/83  "<inputplate_angle>"
  Bus Selector/84 -> Mux/84  "<inputplate_omega>"
  Bus Selector/85 -> Mux/85  "<inputplate_alpha>"
  Bus Selector/86 -> Mux/86  "<efficiency>"
  Bus Selector/87 -> Mux/87  "<efficiency>"
  Bus Selector/88 -> Mux/88  "<diff_front_inputshaft_torque>"
  Bus Selector/89 -> Mux/89  "<diff_rear_inputshaft_torque>"
  Bus Selector/90 -> Mux/90  "<gearbox_outputshaft_angle>"
  Bus Selector/91 -> Mux/91  "<gearbox_outputshaft_omega>"
  Bus Selector/92 -> Mux/92  "<gearbox_outputshaft_alpha>"
  Bus Selector/93 -> Mux/93  "<efficiency>"
  Bus Selector/94 -> Mux/94  "<wheel_front_left_torque>"
  Bus Selector/95 -> Mux/95  "<wheel_front_right_torque>"
  Bus Selector/96 -> Mux/96  "<diff_central_front_outputshaft_angle>"
  Bus Selector/97 -> Mux/97  "<diff_central_front_outputshaft_omega>"
  Bus Selector/98 -> Mux/98  "<diff_central_front_outputshaft_alpha>"
  Bus Selector/99 -> Mux/99  "<efficiency>"
  Bus Selector/100 -> Mux/100  "<wheel_rear_left_torque>"
  Bus Selector/101 -> Mux/101  "<wheel_rear_right_torque>"
  Bus Selector/102 -> Mux/102  "<diff_central_rear_outputshaft_angle>"
  Bus Selector/103 -> Mux/103  "<diff_central_rear_outputshaft_omega>"
  Bus Selector/104 -> Mux/104  "<diff_central_rear_outputshaft_alpha>"
  Bus Selector/105 -> Mux/105  "<front>"
  Bus Selector/106 -> Mux/106  "<rear>"
  Bus Selector/107 -> Mux/107  "<front>"
  Bus Selector/108 -> Mux/108  "<rear>"
  Bus Selector/109 -> Mux/109  "<L1>"
  Bus Selector/110 -> Mux/110  "<L2>"
  Bus Selector/111 -> Mux/111  "<R1>"
  Bus Selector/112 -> Mux/112  "<R2>"
  Bus Selector/113 -> Mux/113  "<Internal_Aero_Activity>"
  Bus Selector/114 -> Mux/114  "<my_scaling>"
  Bus Selector/115 -> Mux/115  "<fx_central_scaling>"
  Bus Selector/116 -> Mux/116  "<fz_front_scaling>"
  Bus Selector/117 -> Mux/117  "<fz_rear_scaling>"
  Bus Selector/118 -> Mux/118  "<fx_front>"
  Bus Selector/119 -> Mux/119  "<fy_front>"
  Bus Selector/120 -> Mux/120  "<fz_front>"
  Bus Selector/121 -> Mux/121  "<fx_rear>"
  Bus Selector/122 -> Mux/122  "<fy_rear>"
  Bus Selector/123 -> Mux/123  "<fz_rear>"
  Bus Selector/124 -> Mux/124  "<fx_center>"
  Bus Selector/125 -> Mux/125  "<fy_center>"
  Bus Selector/126 -> Mux/126  "<fz_center>"
  Bus Selector/127 -> Mux/127  "<mx>"
  Bus Selector/128 -> Mux/128  "<my>"
  Bus Selector/129 -> Mux/129  "<mz>"
  Bus Selector/130 -> Mux/130  "<L1>"
  Bus Selector/131 -> Mux/131  "<L2>"
  Bus Selector/132 -> Mux/132  "<R1>"
  Bus Selector/133 -> Mux/133  "<R2>"
  Bus Selector/134 -> Mux/134  "<L1>"
  Bus Selector/135 -> Mux/135  "<L1>"
  Bus Selector/136 -> Mux/136  "<L2>"
  Bus Selector/137 -> Mux/137  "<L2>"
  Bus Selector/138 -> Mux/138  "<R1>"
  Bus Selector/139 -> Mux/139  "<R1>"
  Bus Selector/140 -> Mux/140  "<R2>"
  Bus Selector/141 -> Mux/141  "<R2>"
  Bus Selector/142 -> Mux/142  "<L1>"
  Bus Selector/143 -> Mux/143  "<L1>"
  Bus Selector/144 -> Mux/144  "<L2>"
  Bus Selector/145 -> Mux/145  "<L2>"
  Bus Selector/146 -> Mux/146  "<R1>"
  Bus Selector/147 -> Mux/147  "<R1>"
  Bus Selector/148 -> Mux/148  "<R2>"
  Bus Selector/149 -> Mux/149  "<R2>"
  Bus Selector/150 -> Mux/150  "<L1>"
  Bus Selector/151 -> Mux/151  "<L1>"
  Bus Selector/152 -> Mux/152  "<L2>"
  Bus Selector/153 -> Mux/153  "<L2>"
  Bus Selector/154 -> Mux/154  "<R1>"
  Bus Selector/155 -> Mux/155  "<R1>"
  Bus Selector/156 -> Mux/156  "<R2>"
  Bus Selector/157 -> Mux/157  "<R2>"
  Bus Selector/158 -> Mux/158  "<L1>"
  Bus Selector/159 -> Mux/159  "<L1>"
  Bus Selector/160 -> Mux/160  "<L2>"
  Bus Selector/161 -> Mux/161  "<L2>"
  Bus Selector/162 -> Mux/162  "<R1>"
  Bus Selector/163 -> Mux/163  "<R1>"
  Bus Selector/164 -> Mux/164  "<R2>"
  Bus Selector/165 -> Mux/165  "<R2>"
  Bus Selector/166 -> Mux/166  "<L1>"
  Bus Selector/167 -> Mux/167  "<L1>"
  Bus Selector/168 -> Mux/168  "<L2>"
  Bus Selector/169 -> Mux/169  "<L2>"
  Bus Selector/170 -> Mux/170  "<R1>"
  Bus Selector/171 -> Mux/171  "<R1>"
  Bus Selector/172 -> Mux/172  "<R2>"
  Bus Selector/173 -> Mux/173  "<R2>"
  Bus Selector/174 -> Mux/174  "<L1>"
  Bus Selector/175 -> Mux/175  "<L1>"
  Bus Selector/176 -> Mux/176  "<L2>"
  Bus Selector/177 -> Mux/177  "<L2>"
  Bus Selector/178 -> Mux/178  "<R1>"
  Bus Selector/179 -> Mux/179  "<R1>"
  Bus Selector/180 -> Mux/180  "<R2>"
  Bus Selector/181 -> Mux/181  "<R2>"
  Bus Selector/182 -> Mux/182  "<front>"
  Bus Selector/183 -> Mux/183  "<front>"
  Bus Selector/184 -> Mux/184  "<rear>"
  Bus Selector/185 -> Mux/185  "<rear>"
  Bus Selector/186 -> Mux/186  "<front>"
  Bus Selector/187 -> Mux/187  "<front>"
  Bus Selector/188 -> Mux/188  "<rear>"
  Bus Selector/189 -> Mux/189  "<rear>"
  Bus Selector/190 -> Mux/190  "<front>"
  Bus Selector/191 -> Mux/191  "<front>"
  Bus Selector/192 -> Mux/192  "<rear>"
  Bus Selector/193 -> Mux/193  "<rear>"
  Bus Selector/194 -> Mux/194  "<front>"
  Bus Selector/195 -> Mux/195  "<front>"
  Bus Selector/196 -> Mux/196  "<rear>"
  Bus Selector/197 -> Mux/197  "<rear>"
  Bus Selector/198 -> Mux/198  "<front>"
  Bus Selector/199 -> Mux/199  "<front>"
  Bus Selector/200 -> Mux/200  "<rear>"
  Bus Selector/201 -> Mux/201  "<rear>"
  Bus Selector/202 -> Mux/202  "<front>"
  Bus Selector/203 -> Mux/203  "<front>"
  Bus Selector/204 -> Mux/204  "<rear>"
  Bus Selector/205 -> Mux/205  "<rear>"
  Bus Selector/206 -> Mux/206  "<front>"
  Bus Selector/207 -> Mux/207  "<front>"
  Bus Selector/208 -> Mux/208  "<rear>"
  Bus Selector/209 -> Mux/209  "<rear>"
  Bus Selector/210 -> Mux/210  "<front>"
  Bus Selector/211 -> Mux/211  "<front>"
  Bus Selector/212 -> Mux/212  "<rear>"
  Bus Selector/213 -> Mux/213  "<rear>"
  Bus Selector/214 -> Mux/214  "<front>"
  Bus Selector/215 -> Mux/215  "<front>"
  Bus Selector/216 -> Mux/216  "<rear>"
  Bus Selector/217 -> Mux/217  "<rear>"
  Bus Selector/218 -> Mux/218  "<front>"
  Bus Selector/219 -> Mux/219  "<front>"
  Bus Selector/220 -> Mux/220  "<rear>"
  Bus Selector/221 -> Mux/221  "<rear>"
  Bus Selector/222 -> Mux/222  "<L1>"
  Bus Selector/223 -> Mux/223  "<L1>"
  Bus Selector/224 -> Mux/224  "<L1>"
  Bus Selector/225 -> Mux/225  "<L1>"
  Bus Selector/226 -> Mux/226  "<L1>"
  Bus Selector/227 -> Mux/227  "<L1>"
  Bus Selector/228 -> Mux/228  "<L1>"
  Bus Selector/229 -> Mux/229  "<L1>"
  Bus Selector/230 -> Mux/230  "<L1>"
  Bus Selector/231 -> Mux/231  "<L1>"
  Bus Selector/232 -> Mux/232  "<L1>"
  Bus Selector/233 -> Mux/233  "<L1>"
  Bus Selector/234 -> Mux/234  "<L2>"
  Bus Selector/235 -> Mux/235  "<L2>"
  Bus Selector/236 -> Mux/236  "<L2>"
  Bus Selector/237 -> Mux/237  "<L2>"
  Bus Selector/238 -> Mux/238  "<L2>"
  Bus Selector/239 -> Mux/239  "<L2>"
  Bus Selector/240 -> Mux/240  "<L2>"
  Bus Selector/241 -> Mux/241  "<L2>"
  Bus Selector/242 -> Mux/242  "<L2>"
  Bus Selector/243 -> Mux/243  "<L2>"
  Bus Selector/244 -> Mux/244  "<L2>"
  Bus Selector/245 -> Mux/245  "<L2>"
  Bus Selector/246 -> Mux/246  "<R1>"
  Bus Selector/247 -> Mux/247  "<R1>"
  Bus Selector/248 -> Mux/248  "<R1>"
  Bus Selector/249 -> Mux/249  "<R1>"
  Bus Selector/250 -> Mux/250  "<R1>"
  Bus Selector/251 -> Mux/251  "<R1>"
  Bus Selector/252 -> Mux/252  "<R1>"
  Bus Selector/253 -> Mux/253  "<R1>"
  Bus Selector/254 -> Mux/254  "<R1>"
  Bus Selector/255 -> Mux/255  "<R1>"
  Bus Selector/256 -> Mux/256  "<R1>"
  Bus Selector/257 -> Mux/257  "<R1>"
  Bus Selector/258 -> Mux/258  "<R2>"
  Bus Selector/259 -> Mux/259  "<R2>"
  Bus Selector/260 -> Mux/260  "<R2>"
  Bus Selector/261 -> Mux/261  "<R2>"
  Bus Selector/262 -> Mux/262  "<R2>"
  Bus Selector/263 -> Mux/263  "<R2>"
  Bus Selector/264 -> Mux/264  "<R2>"
  Bus Selector/265 -> Mux/265  "<R2>"
  Bus Selector/266 -> Mux/266  "<R2>"
  Bus Selector/267 -> Mux/267  "<R2>"
  Bus Selector/268 -> Mux/268  "<R2>"
  Bus Selector/269 -> Mux/269  "<R2>"
  Bus Selector/270 -> Mux/270  "<X>"
  Bus Selector/271 -> Mux/271  "<Y>"
  Bus Selector/272 -> Mux/272  "<Z>"
  Bus Selector/273 -> Mux/273  "<X>"
  Bus Selector/274 -> Mux/274  "<Y>"
  Bus Selector/275 -> Mux/275  "<Z>"
  Bus Selector/276 -> Mux/276  "<X>"
  Bus Selector/277 -> Mux/277  "<Y>"
  Bus Selector/278 -> Mux/278  "<Z>"
  Bus Selector/279 -> Mux/279  "<X>"
  Bus Selector/280 -> Mux/280  "<Y>"
  Bus Selector/281 -> Mux/281  "<Z>"
  Bus Selector/282 -> Mux/282  "<X>"
  Bus Selector/283 -> Mux/283  "<Y>"
  Bus Selector/284 -> Mux/284  "<X>"
  Bus Selector/285 -> Mux/285  "<Y>"
  Bus Selector/286 -> Mux/286  "<force>"
  Bus Selector/287 -> Mux/287  "<torque>"
  Bus Selector/288 -> Mux/288  "<torque>"
  Bus Selector/289 -> Mux/289  "<motor_torque>"
  Bus Selector/290 -> Mux/290  "<auxiliary_steering_torque>"
  Bus Selector/291 -> Mux/291  "<eps_map>"
  Bus Selector/292 -> Mux/292  "<Internal_mass_activation>"
  Bus Selector/293 -> Mux/293  "<External_mass>"
  Bus Selector/294 -> Mux/294  "<efficiency>"
  Bus Selector/295 -> Mux/295  "<transmission_ratio>"
  Bus Selector/296 -> Mux/296  "<diff_central_inputshaft_torque>"
  Bus Selector/297 -> Mux/297  "<clutch_outputplate_angle>"
  Bus Selector/298 -> Mux/298  "<clutch_outputplate_omega>"
  Bus Selector/299 -> Mux/299  "<clutch_outputplate_alpha>"
  Bus Selector/300 -> Mux/300  "<automatic_gearbox_shifting_mode>"
  Bus Selector/301 -> Mux/301  "<manual_shifting_activity>"
  Bus Selector/302 -> Mux/302  "<sequential_shifting_activity>"
  Bus Selector/303 -> Mux/303  "<gear_upshift>"
  Bus Selector/304 -> Mux/304  "<gear_downshift>"

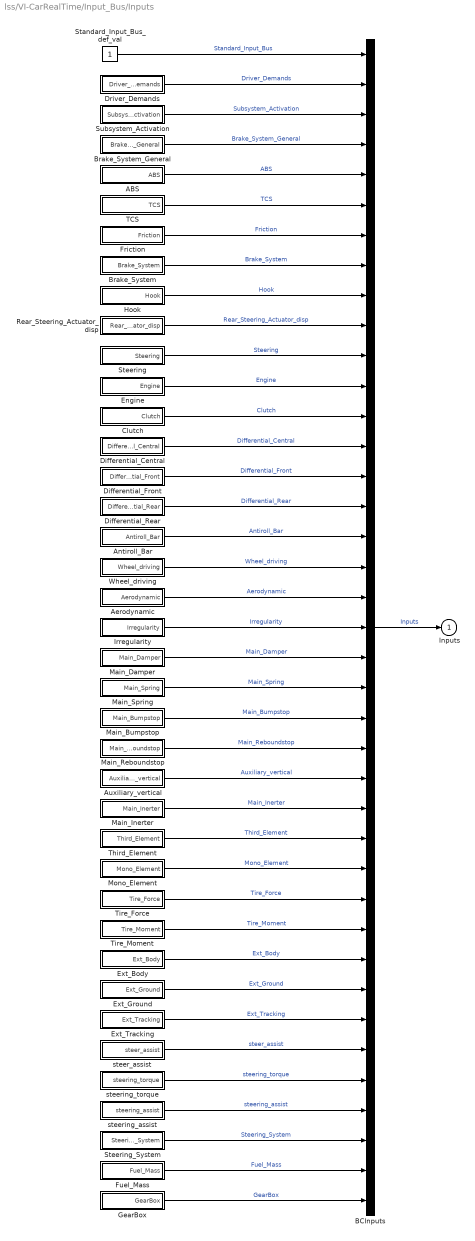
== system lss/VI-CarRealTime/Input_Bus/Inputs ==
  ABS : Subsystem
  Aerodynamic : Subsystem
  Antiroll_Bar : Subsystem
  Auxiliary_vertical : Subsystem
  BCInputs : BusCreator  Inputs=39
  Brake_System : Subsystem
  Brake_System_General : Subsystem
  Clutch : Subsystem
  Differential_Central : Subsystem
  Differential_Front : Subsystem
  Differential_Rear : Subsystem
  Driver_Demands : Subsystem
  Engine : Subsystem
  Ext_Body : Subsystem
  Ext_Ground : Subsystem
  Ext_Tracking : Subsystem
  Friction : Subsystem
  Fuel_Mass : Subsystem
  GearBox : Subsystem
  Hook : Subsystem
  Irregularity : Subsystem
  Main_Bumpstop : Subsystem
  Main_Damper : Subsystem
  Main_Inerter : Subsystem
  Main_Reboundstop : Subsystem
  Main_Spring : Subsystem
  Mono_Element : Subsystem
  Rear_Steering_Actuator_disp : Subsystem
  Standard_Input_Bus_def_val : Constant
  Steering : Subsystem
  Steering_System : Subsystem
  Subsystem_Activation : Subsystem
  TCS : Subsystem
  Third_Element : Subsystem
  Tire_Force : Subsystem
  Tire_Moment : Subsystem
  Wheel_driving : Subsystem
  steer_assist : Subsystem
  steering_assist : Subsystem
  steering_torque : Subsystem
  Inputs : Outport
  wires:
  BCInputs/1 -> Inputs/1  "Inputs"
  Standard_Input_Bus_def_val/1 -> BCInputs/1  "Standard_Input_Bus"
  Driver_Demands/1(Driver_Demands) -> BCInputs/2  "Driver_Demands"
  Subsystem_Activation/1(Subsystem_Activation) -> BCInputs/3  "Subsystem_Activation"
  Brake_System_General/1(Brake_System_General) -> BCInputs/4  "Brake_System_General"
  ABS/1(ABS) -> BCInputs/5  "ABS"
  TCS/1(TCS) -> BCInputs/6  "TCS"
  Friction/1(Friction) -> BCInputs/7  "Friction"
  Brake_System/1(Brake_System) -> BCInputs/8  "Brake_System"
  Hook/1(Hook) -> BCInputs/9  "Hook"
  Rear_Steering_Actuator_disp/1(Rear_Steering_Actuator_disp) -> BCInputs/10  "Rear_Steering_Actuator_disp"
  Steering/1(Steering) -> BCInputs/11  "Steering"
  Engine/1(Engine) -> BCInputs/12  "Engine"
  Clutch/1(Clutch) -> BCInputs/13  "Clutch"
  Differential_Central/1(Differential_Central) -> BCInputs/14  "Differential_Central"
  Differential_Front/1(Differential_Front) -> BCInputs/15  "Differential_Front"
  Differential_Rear/1(Differential_Rear) -> BCInputs/16  "Differential_Rear"
  Antiroll_Bar/1(Antiroll_Bar) -> BCInputs/17  "Antiroll_Bar"
  Wheel_driving/1(Wheel_driving) -> BCInputs/18  "Wheel_driving"
  Aerodynamic/1(Aerodynamic) -> BCInputs/19  "Aerodynamic"
  Irregularity/1(Irregularity) -> BCInputs/20  "Irregularity"
  Main_Damper/1(Main_Damper) -> BCInputs/21  "Main_Damper"
  Main_Spring/1(Main_Spring) -> BCInputs/22  "Main_Spring"
  Main_Bumpstop/1(Main_Bumpstop) -> BCInputs/23  "Main_Bumpstop"
  Main_Reboundstop/1(Main_Reboundstop) -> BCInputs/24  "Main_Reboundstop"
  Auxiliary_vertical/1(Auxiliary_vertical) -> BCInputs/25  "Auxiliary_vertical"
  Main_Inerter/1(Main_Inerter) -> BCInputs/26  "Main_Inerter"
  Third_Element/1(Third_Element) -> BCInputs/27  "Third_Element"
  Mono_Element/1(Mono_Element) -> BCInputs/28  "Mono_Element"
  Tire_Force/1(Tire_Force) -> BCInputs/29  "Tire_Force"
  Tire_Moment/1(Tire_Moment) -> BCInputs/30  "Tire_Moment"
  Ext_Body/1(Ext_Body) -> BCInputs/31  "Ext_Body"
  Ext_Ground/1(Ext_Ground) -> BCInputs/32  "Ext_Ground"
  Ext_Tracking/1(Ext_Tracking) -> BCInputs/33  "Ext_Tracking"
  steer_assist/1(steer_assist) -> BCInputs/34  "steer_assist"
  steering_torque/1(steering_torque) -> BCInputs/35  "steering_torque"
  steering_assist/1(steering_assist) -> BCInputs/36  "steering_assist"
  Steering_System/1(Steering_System) -> BCInputs/37  "Steering_System"
  Fuel_Mass/1(Fuel_Mass) -> BCInputs/38  "Fuel_Mass"
  GearBox/1(GearBox) -> BCInputs/39  "GearBox"
